simulink model "TenseSimIntepretted"  (R2022b)
settings: Solver=daessc  StartTime=0.0  StopTime=0.3  RelTol=1e-3
StartFcn:
  | myMech = tenseMech();
settings Model: SimulationMode=accelerator  Creator=theko  LastModifiedBy=theko

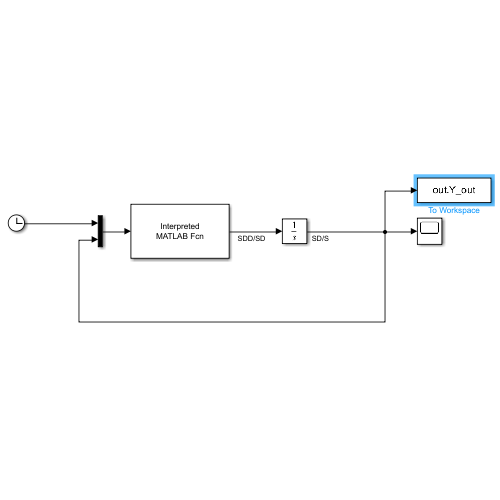
[thumbnail: Simulink's stored preview of the top-level diagram]
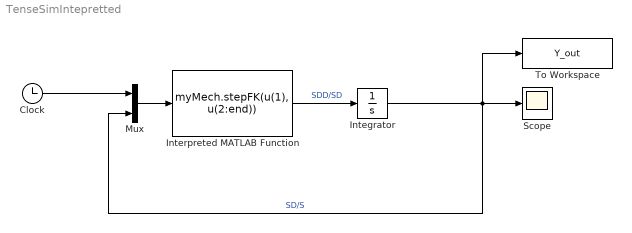
== system TenseSimIntepretted ==
  Clock : Clock
  Integrator : Integrator  InitialCondition=myMech.Y_sim
  Interpreted MATLAB Function : MATLABFcn  MATLABFcn=myMech.stepFK(u(1), u(2:end))  OutputDimensions=84  OutputSignalType=real
  Mux : Mux  Inputs=2
  Scope : Scope
  To Workspace : ToWorkspace  VariableName=Y_out  SaveFormat=Structure With Time  SampleTime=-1
  wires:
  Interpreted MATLAB Function/1 -> Integrator/1  "SDD/SD"
  Mux/1 -> Interpreted MATLAB Function/1
  Clock/1 -> Mux/1
  Integrator/1 -> To Workspace/1, Scope/1, Mux/2  "SD/S"
